simulink model "VCM20_TCon"  (R2021b)
settings: Solver=ode1  StartTime=0.0  StopTime=Inf  FixedStep=0.001  RelTol=1e-3
PostLoadFcn:
  | , if any(exist('dsrtsu_mdlpostloadfcn', 'file') ~= 0), dsrtsu_mdlpostloadfcn('Execute', bdroot); end,
values from neighbouring files (symbols this model uses):
  gear_f = 14.45    [VehicleParamsFEM20_Gear17.m]
  Rwf = 18*(25.4/1000)/2    (= 0.2286)    [VehicleParamsFEM20_Gear17.m]
libraries: rtican x62, dspstat3 x9, simulink x8, rti1401lib_dio_type4 x4, rti1401lib_adc_type4 x4
(part 5 of 12)

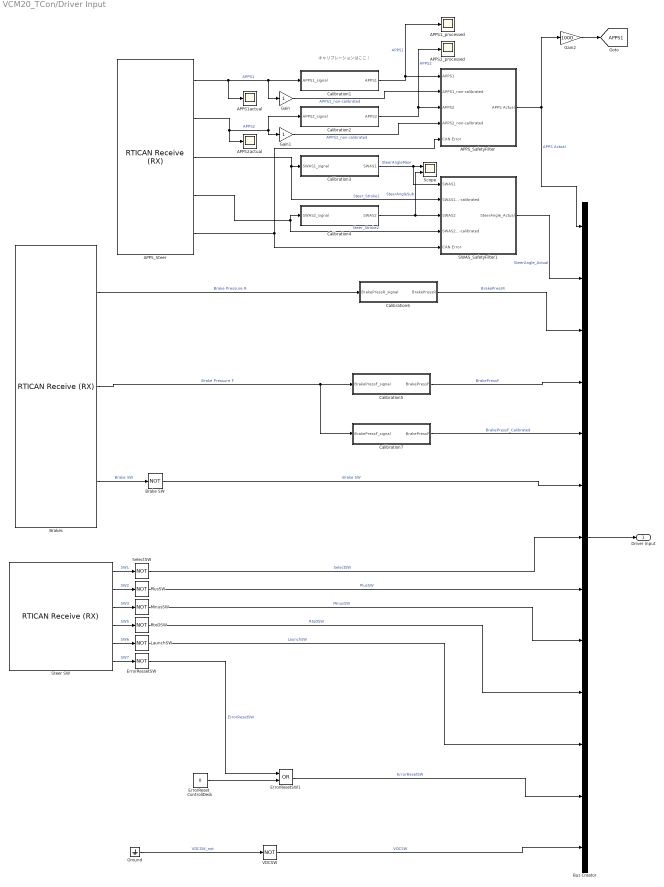
== system VCM20_TCon/Driver Input ==
  note: キャリブレーションはここ！
  APPS1_processed : Scope
  APPS1actual : Scope
  APPS2_processed : Scope
  APPS2actual : Scope
  APPS_SafetyFilter : Subsystem
  APPS_Steer : rtican/RTICAN Receive (RX)   Reserved1=[]  Reserved2=[]  Reserved3=[]  Reserved4=[]  SfcnMessage=[]  Msg_Struct=[]  BoardTypeNo=[]  BoardNo=[]  ChannelNo=[]  Parameters=[]  DialogFcn=[]  UnitName=[]  Revision=[]  UnitValues=[]  DSProperties=struct('RTI',struct('Version',uint32(5),'BlockType',struct('isSLSource',uint8(1),'isSLSink',uint8(1),'isHWSource',uint8(0),'isHWSink',uint8(0),'isSetup',uint8(0),'isInline',uint8(1),'isNonInline',uint8(0),'isInterrupt',uint8(0),'isChannelwise',uint8(0)),'IOBoardType','RTICAN','UnitType','MESSAGE','Identifier','RX','DialogType','MSVC','BlockSet','RTICAN','SlaveProcessor','CAN'))  RTIBlockInterface=struct('OutputPortsWidth',int32([1 1 1 1 1]),'OutputPortsActive',[1 1 1 1 1],'OutputPortsName',{{'APPS1','APPS2','Steer_Stroke1','Steer_Stroke2',['RX status']}},'OutputPortsDataType',{{'SS_DOUBLE','SS_DOUBLE','SS_DOUBLE','SS_DOUBLE','SS_DOUBLE'}},'OutputPortsLabel',{{'APPS1','APPS2','Steer_Stroke1','Steer_Stroke2',''}},'OutputPortsLabelMode','ON','InputPortsWidth',int32(0),'InputPortsActive',0,'DialogFcn','rtican_message_interface_gui','BlockDisplay',{{'','center'}},'IconTransparency','on','ParameterTunableNames',{{}},'InitLevel',3,'BlockName',struct('Token',{{'APPS_Steer'}}),'SampleTime',{{0.01}},'TriggerPort',{{'none'}},'EnablePort',{{'none'}})  RTIBlockParameters=struct('BoardTypeNo',{{1,'OFF',[]}},'BoardNo',{{3,'ON',[1 16]}},'ChannelNo',{{2,'ON',[1 2]}},'Parameters',{{struct('DataFileSupport',struct('DataFileSelectedMaster',0,'DataFileSelectedLocal',0,'DataFileName',['<no datafile support>|'],'DataFileDate','','SelectedFile',['<no file selected>']),'Options',struct('StatusSelected',1,'TimeSelected',0,'DeltaTimeSelected',0,'BytePortSelected',0,'MessageLengthSelected',0,'TriggerPort',struct('Selected',0,'TriggerType',0),'UserCoding',struct('Selected',0,'InterfaceFile','UserDecodingFile','FcnName','UserDecodeFcn','InportSelected',0,'InportWidth',1,'OutportSelected',0,'OutportWidth',1),'EnablePortSelected',0,'SignalOnPortnameSelected',1,'UseRXService',0),'Message',struct('MsgOnBlocknameSelected',1,'MsgName','APPS_Steer','MsgIdFormat',0,'MsgId',513,'MsgLength',8,'NumSignals',4,'SampleTime',0.01,'Signal',struct('SgnName',{'APPS1','APPS2','Steer_Stroke1','Steer_Stroke2'},'SgnStartBit',{0,16,32,48},'SgnLength',{16,16,16,16},'SgnType',{0,0,0,0},'ModeValue',{-1,-1,-1,-1},'DataType',{0,0,0,0},'ByteLayout',{0,0,0,0},'Factor',{1,1,1,1},'Offset',{0,0,0,0},'SgnComment',{{''},{''},{''},{''}},'SgnUnit',{'','','',''},'Min',{0,0,0,0},'Max',{0,0,0,0},'SLDataType',{'SS_DOUBLE','SS_DOUBLE','SS_DOUBLE','SS_DOUBLE'}),'MsgIdNumFormat',1,'MsgComment',{{''}}),'Version',1.2,'general',struct('isFromLib',0)),'OFF',[]}},'GroupId',{{struct('Group',{{'RTICAN'}},'No',6,'Behavior',{{'NAMECHANGE'}},'BlockType',{{'SINK'}},'NameChangeFlag',0),'OFF',[]}},'SFcnRTICANMessage',{{struct('MsgType','RX','SFcnPortType','Scalar','MsgName','APPS_Steer','MsgIdFormat','STD','MsgId',513,'MsgLength',8,'NumSignals',4,'SampleTime',0.01,'Signal',struct('SgnName',{'APPS1','APPS2','Steer_Stroke1','Steer_Stroke2'},'SgnStartBit',{0,16,32,48},'SgnLength',{16,16,16,16},'SgnType',{'standard','standard','standard','standard'},'ModeValue',{-1,-1,-1,-1},'DataType',{['unsigned int'],['unsigned int'],['unsigned int'],['unsigned int']},'ByteLayout',{['little endian'],['little endian'],['little endian'],['little endian']},'Factor',{1,1,1,1},'Offset',{0,0,0,0},'SLDataType',{'SS_DOUBLE','SS_DOUBLE','SS_DOUBLE','SS_DOUBLE'}),'StatusSelected','yes','TimeSelected','no','DeltaTimeSelected','no','BytePortSelected','no','MessageLengthSelected','no','TriggerPort',struct('Selected','no','TriggerType',0),'UserCoding',struct('Selected','no','InterfaceFile','UserDecodingFile','FcnName','UserDecodeFcn','InportSelected','no','InportWidth',1,'OutportSelected','no','OutportWidth',1),'EnablePortSelected','no','UseRXService','no','BoardType','DS1','BoardNo',3,'ControllerNo',2),'OFF',[]}},'TLCFileName',{{'rtican_rx_message','OFF',[]}})  RTISFcnParameters=struct('SFcnRTICANMessage','struct','TLCFileName','char')  RTIBlockParaDefault=struct('BoardTypeNo',4302,'BoardNo',1,'ChannelNo',1,'Parameters',struct('DataFileSupport',struct('DataFileSelectedMaster',0,'DataFileSelectedLocal',0,'DataFileName','','DataFileDate','','SelectedFile',['<no file selected>']),'Options',struct('StatusSelected',1,'TimeSelected',1,'DeltaTimeSelected',1,'BytePortSelected',0,'MessageLengthSelected',0,'TriggerPort',struct('Selected',0,'TriggerType','rising'),'UserCoding',struct('Selected',0,'InterfaceFile','UserDecodingFile','FcnName','UserDecodeFcn','InportSelected',0,'InportWidth',1,'OutportSelected',0,'OutportWidth',1),'EnablePortSelected',0,'SignalOnPortnameSelected',1,'UseRXService',0),'Message',struct('MsgOnBlocknameSelected',0,'MsgName',['RX Message'],'MsgIdFormat',0,'MsgId',100,'MsgLength',8,'NumSignals',1,'SampleTime',-1,'Signal',struct('SgnName',['RX signal'],'SgnStartBit',0,'SgnLength',8,'SgnType',0,'ModeValue',-1,'DataType',0,'SLDataType','SS_DOUBLE','ByteLayout',0,'Factor',1,'Offset',0,'Min',0,'Max',255,'SgnComment',{{}},'SgnUnit',''),'MsgIdNumFormat',0,'MsgComment',{{''}}),'Version',1.2,'general',struct('isFromLib',1)),'GroupId',struct('Group',{{'RTICAN'}},'No',1,'Behavior',{{'NAMECHANGE'}},'BlockType',{{'SINK'}},'NameChangeFlag',0),'SFcnRTICANMessage',struct('MsgType','RX','MsgName',['RX Message'],'MsgIdFormat','STD','MsgId',100,'MsgLength',8,'NumSignals',1,'SampleTime',-1,'Signal',struct('SgnName',['RX signal'],'SgnStartBit',0,'SgnLength',8,'SgnType','standard','ModeValue',-1,'DataType',['unsigned int'],'ByteLayout',['little endian'],'SLDataType','SS_DOUBLE','Factor',1,'Offset',0),'StatusSelected','yes','TimeSelected','yes','DeltaTimeSelected','yes','BytePortSelected','no','MessageLengthSelected','no','EnablePortSelected','no','UserCoding',struct('Selected','no','InterfaceFile','UserDecodingFile','FcnName','UserDecodeFcn','InportSelected','no','InportWidth',1,'OutportSelected','no','OutportWidth',1),'TriggerPort',struct('Selected','no','TriggerType','rising'),'UseRXService','no','BoardType','DS4302','BoardNo',1,'ControllerNo',1,'SFcnPortType','Scalar'),'TLCFileName','rtican_rx_message')
      settings: AttributesFormatString=Group Id: RTICAN6\n  SourceProductName=dSPACE RTI CAN Blockset
  Brake SW : Logic  Operator=NOT  IconShape=distinctive  AllPortsSameDT=off  OutDataTypeStr=boolean
  Brakes : rtican/RTICAN Receive (RX)   Reserved1=[]  Reserved2=[]  Reserved3=[]  Reserved4=[]  SfcnMessage=[]  Msg_Struct=[]  BoardTypeNo=[]  BoardNo=[]  ChannelNo=[]  Parameters=[]  DialogFcn=[]  UnitName=[]  Revision=[]  UnitValues=[]  DSProperties=struct('RTI',struct('Version',uint32(5),'BlockType',struct('isSLSource',uint8(1),'isSLSink',uint8(1),'isHWSource',uint8(0),'isHWSink',uint8(0),'isSetup',uint8(0),'isInline',uint8(1),'isNonInline',uint8(0),'isInterrupt',uint8(0),'isChannelwise',uint8(0)),'IOBoardType','RTICAN','UnitType','MESSAGE','Identifier','RX','DialogType','MSVC','BlockSet','RTICAN','SlaveProcessor','CAN'))  RTIBlockInterface=struct('OutputPortsWidth',int32([1 1 1]),'OutputPortsActive',[1 1 1],'OutputPortsName',{{['Brake Pressure R'],['Brake Pressure F'],['Brake SW']}},'OutputPortsDataType',{{'SS_DOUBLE','SS_DOUBLE','SS_DOUBLE'}},'OutputPortsLabel',{{['Brake Pressure R'],['Brake Pressure F'],['Brake SW']}},'OutputPortsLabelMode','ON','InputPortsWidth',int32(0),'InputPortsActive',0,'DialogFcn','rtican_message_interface_gui','BlockDisplay',{{'','center'}},'IconTransparency','on','ParameterTunableNames',{{}},'InitLevel',3,'BlockName',struct('Token',{{'Brakes'}}),'SampleTime',{{0.01}},'TriggerPort',{{'none'}},'EnablePort',{{'none'}})  RTIBlockParameters=struct('BoardTypeNo',{{1,'OFF',[]}},'BoardNo',{{3,'ON',[1 16]}},'ChannelNo',{{2,'ON',[1 2]}},'Parameters',{{struct('DataFileSupport',struct('DataFileSelectedMaster',0,'DataFileSelectedLocal',0,'DataFileName',['<no datafile support>|'],'DataFileDate','','SelectedFile',['<no file selected>']),'Options',struct('StatusSelected',0,'TimeSelected',0,'DeltaTimeSelected',0,'BytePortSelected',0,'MessageLengthSelected',0,'TriggerPort',struct('Selected',0,'TriggerType',0),'UserCoding',struct('Selected',0,'InterfaceFile','UserDecodingFile','FcnName','UserDecodeFcn','InportSelected',0,'InportWidth',1,'OutportSelected',0,'OutportWidth',1),'EnablePortSelected',0,'SignalOnPortnameSelected',1,'UseRXService',0),'Message',struct('MsgOnBlocknameSelected',1,'MsgName','Brakes','MsgIdFormat',0,'MsgId',514,'MsgLength',8,'NumSignals',3,'SampleTime',0.01,'Signal',struct('SgnName',{['Brake Pressure R'],['Brake Pressure F'],['Brake SW']},'SgnStartBit',{0,16,32},'SgnLength',{16,16,8},'SgnType',{0,0,0},'ModeValue',{-1,-1,-1},'DataType',{0,0,0},'ByteLayout',{0,0,0},'Factor',{1,1,1},'Offset',{0,0,0},'SgnComment',{{''},{''},{''}},'SgnUnit',{'','',''},'Min',{0,0,0},'Max',{0,0,0},'SLDataType',{'SS_DOUBLE','SS_DOUBLE','SS_DOUBLE'}),'MsgIdNumFormat',1,'MsgComment',{{''}}),'Version',1.2,'general',struct('isFromLib',0)),'OFF',[]}},'GroupId',{{struct('Group',{{'RTICAN'}},'No',6,'Behavior',{{'NAMECHANGE'}},'BlockType',{{'SINK'}},'NameChangeFlag',0),'OFF',[]}},'SFcnRTICANMessage',{{struct('MsgType','RX','SFcnPortType','Scalar','MsgName','Brakes','MsgIdFormat','STD','MsgId',514,'MsgLength',8,'NumSignals',3,'SampleTime',0.01,'Signal',struct('SgnName',{['Brake Pressure R'],['Brake Pressure F'],['Brake SW']},'SgnStartBit',{0,16,32},'SgnLength',{16,16,8},'SgnType',{'standard','standard','standard'},'ModeValue',{-1,-1,-1},'DataType',{['unsigned int'],['unsigned int'],['unsigned int']},'ByteLayout',{['little endian'],['little endian'],['little endian']},'Factor',{1,1,1},'Offset',{0,0,0},'SLDataType',{'SS_DOUBLE','SS_DOUBLE','SS_DOUBLE'}),'StatusSelected','no','TimeSelected','no','DeltaTimeSelected','no','BytePortSelected','no','MessageLengthSelected','no','TriggerPort',struct('Selected','no','TriggerType',0),'UserCoding',struct('Selected','no','InterfaceFile','UserDecodingFile','FcnName','UserDecodeFcn','InportSelected','no','InportWidth',1,'OutportSelected','no','OutportWidth',1),'EnablePortSelected','no','UseRXService','no','BoardType','DS1','BoardNo',3,'ControllerNo',2),'OFF',[]}},'TLCFileName',{{'rtican_rx_message','OFF',[]}})  RTISFcnParameters=struct('SFcnRTICANMessage','struct','TLCFileName','char')  RTIBlockParaDefault=struct('BoardTypeNo',4302,'BoardNo',1,'ChannelNo',1,'Parameters',struct('DataFileSupport',struct('DataFileSelectedMaster',0,'DataFileSelectedLocal',0,'DataFileName','','DataFileDate','','SelectedFile',['<no file selected>']),'Options',struct('StatusSelected',1,'TimeSelected',1,'DeltaTimeSelected',1,'BytePortSelected',0,'MessageLengthSelected',0,'TriggerPort',struct('Selected',0,'TriggerType','rising'),'UserCoding',struct('Selected',0,'InterfaceFile','UserDecodingFile','FcnName','UserDecodeFcn','InportSelected',0,'InportWidth',1,'OutportSelected',0,'OutportWidth',1),'EnablePortSelected',0,'SignalOnPortnameSelected',1,'UseRXService',0),'Message',struct('MsgOnBlocknameSelected',0,'MsgName',['RX Message'],'MsgIdFormat',0,'MsgId',100,'MsgLength',8,'NumSignals',1,'SampleTime',-1,'Signal',struct('SgnName',['RX signal'],'SgnStartBit',0,'SgnLength',8,'SgnType',0,'ModeValue',-1,'DataType',0,'SLDataType','SS_DOUBLE','ByteLayout',0,'Factor',1,'Offset',0,'Min',0,'Max',255,'SgnComment',{{}},'SgnUnit',''),'MsgIdNumFormat',0,'MsgComment',{{''}}),'Version',1.2,'general',struct('isFromLib',1)),'GroupId',struct('Group',{{'RTICAN'}},'No',1,'Behavior',{{'NAMECHANGE'}},'BlockType',{{'SINK'}},'NameChangeFlag',0),'SFcnRTICANMessage',struct('MsgType','RX','MsgName',['RX Message'],'MsgIdFormat','STD','MsgId',100,'MsgLength',8,'NumSignals',1,'SampleTime',-1,'Signal',struct('SgnName',['RX signal'],'SgnStartBit',0,'SgnLength',8,'SgnType','standard','ModeValue',-1,'DataType',['unsigned int'],'ByteLayout',['little endian'],'SLDataType','SS_DOUBLE','Factor',1,'Offset',0),'StatusSelected','yes','TimeSelected','yes','DeltaTimeSelected','yes','BytePortSelected','no','MessageLengthSelected','no','EnablePortSelected','no','UserCoding',struct('Selected','no','InterfaceFile','UserDecodingFile','FcnName','UserDecodeFcn','InportSelected','no','InportWidth',1,'OutportSelected','no','OutportWidth',1),'TriggerPort',struct('Selected','no','TriggerType','rising'),'UseRXService','no','BoardType','DS4302','BoardNo',1,'ControllerNo',1,'SFcnPortType','Scalar'),'TLCFileName','rtican_rx_message')
      settings: AttributesFormatString=Group Id: RTICAN6\n  SourceProductName=dSPACE RTI CAN Blockset
  Bus Creator : BusCreator  Inputs=13
  Calibration1 : Subsystem
  Calibration2 : Subsystem
  Calibration3 : Subsystem
  Calibration4 : Subsystem
  Calibration5 : Subsystem
  Calibration6 : Subsystem
  Calibration7 : Subsystem
  ErrorResetSW1 : Logic  Operator=OR  AllPortsSameDT=off  OutDataTypeStr=boolean
  ErrorReset_ControllDesk : Constant  Value=0
  ErrorRessetSW : Logic  Operator=NOT  IconShape=distinctive  AllPortsSameDT=off  OutDataTypeStr=boolean
  Gain : Gain
  Gain1 : Gain
  Gain2 : Gain  Gain=1000
  Ground : Ground
  LaunchSW : Logic  Operator=NOT  IconShape=distinctive  AllPortsSameDT=off  OutDataTypeStr=boolean
  MinusSW : Logic  Operator=NOT  IconShape=distinctive  AllPortsSameDT=off  OutDataTypeStr=boolean
  PlusSW : Logic  Operator=NOT  IconShape=distinctive  AllPortsSameDT=off  OutDataTypeStr=boolean
  RtoDSW : Logic  Operator=NOT  IconShape=distinctive  AllPortsSameDT=off  OutDataTypeStr=boolean
  SWAS_SafetyFilter1 : Subsystem
  Scope : Scope  NumInputPorts=2
  SelectSW : Logic  Operator=NOT  IconShape=distinctive  AllPortsSameDT=off  OutDataTypeStr=boolean
  Steer SW : rtican/RTICAN Receive (RX)   Reserved1=[]  Reserved2=[]  Reserved3=[]  Reserved4=[]  SfcnMessage=[]  Msg_Struct=[]  BoardTypeNo=[]  BoardNo=[]  ChannelNo=[]  Parameters=[]  DialogFcn=[]  UnitName=[]  Revision=[]  UnitValues=[]  DSProperties=struct('RTI',struct('Version',uint32(5),'BlockType',struct('isSLSource',uint8(1),'isSLSink',uint8(1),'isHWSource',uint8(0),'isHWSink',uint8(0),'isSetup',uint8(0),'isInline',uint8(1),'isNonInline',uint8(0),'isInterrupt',uint8(0),'isChannelwise',uint8(0)),'IOBoardType','RTICAN','UnitType','MESSAGE','Identifier','RX','DialogType','MSVC','BlockSet','RTICAN','SlaveProcessor','CAN'))  RTIBlockInterface=struct('OutputPortsWidth',int32([1 1 1 1 1 1]),'OutputPortsActive',[1 1 1 1 1 1],'OutputPortsName',{{'SW1','SW2','SW3','SW5','SW6','SW7'}},'OutputPortsDataType',{{'SS_DOUBLE','SS_DOUBLE','SS_DOUBLE','SS_DOUBLE','SS_DOUBLE','SS_DOUBLE'}},'OutputPortsLabel',{{'SW1','SW2','SW3','SW5','SW6','SW7'}},'OutputPortsLabelMode','ON','InputPortsWidth',int32(0),'InputPortsActive',0,'DialogFcn','rtican_message_interface_gui','BlockDisplay',{{'','center'}},'IconTransparency','on','ParameterTunableNames',{{}},'InitLevel',3,'BlockName',struct('Token',{{'Brakes'}}),'SampleTime',{{0.1}},'TriggerPort',{{'none'}},'EnablePort',{{'none'}})  RTIBlockParameters=struct('BoardTypeNo',{{1,'OFF',[]}},'BoardNo',{{1,'ON',[1 16]}},'ChannelNo',{{1,'ON',[1 2]}},'Parameters',{{struct('DataFileSupport',struct('DataFileSelectedMaster',0,'DataFileSelectedLocal',0,'DataFileName',['<no datafile support>|'],'DataFileDate','','SelectedFile',['<no file selected>']),'Options',struct('StatusSelected',0,'TimeSelected',0,'DeltaTimeSelected',0,'BytePortSelected',0,'MessageLengthSelected',0,'TriggerPort',struct('Selected',0,'TriggerType',0),'UserCoding',struct('Selected',0,'InterfaceFile','UserDecodingFile','FcnName','UserDecodeFcn','InportSelected',0,'InportWidth',1,'OutportSelected',0,'OutportWidth',1),'EnablePortSelected',0,'SignalOnPortnameSelected',1,'UseRXService',0),'Message',struct('MsgOnBlocknameSelected',1,'MsgName',['Steer SW'],'MsgIdFormat',0,'MsgId',512,'MsgLength',1,'NumSignals',6,'SampleTime',0.1,'Signal',struct('SgnName',{'SW1','SW2','SW3','SW5','SW6','SW7'},'SgnStartBit',{0,1,2,3,4,5},'SgnLength',{1,1,1,1,1,1},'SgnType',{0,0,0,0,0,0},'ModeValue',{-1,-1,-1,-1,-1,-1},'DataType',{0,0,0,0,0,0},'ByteLayout',{0,0,0,0,0,0},'Factor',{1,1,1,1,1,1},'Offset',{0,0,0,0,0,0},'SgnComment',{{''},{''},{''},{''},{''},{''}},'SgnUnit',{'','','','','',''},'Min',{0,0,0,0,0,0},'Max',{0,0,0,0,0,0},'SLDataType',{'SS_DOUBLE','SS_DOUBLE','SS_DOUBLE','SS_DOUBLE','SS_DOUBLE','SS_DOUBLE'}),'MsgIdNumFormat',1,'MsgComment',{{''}}),'Version',1.2,'general',struct('isFromLib',0)),'OFF',[]}},'GroupId',{{struct('Group',{{'RTICAN'}},'No',1,'Behavior',{{'NAMECHANGE'}},'BlockType',{{'SINK'}},'NameChangeFlag',0),'OFF',[]}},'SFcnRTICANMessage',{{struct('MsgType','RX','SFcnPortType','Scalar','MsgName',['Steer SW'],'MsgIdFormat','STD','MsgId',512,'MsgLength',1,'NumSignals',6,'SampleTime',0.1,'Signal',struct('SgnName',{'SW1','SW2','SW3','SW5','SW6','SW7'},'SgnStartBit',{0,1,2,3,4,5},'SgnLength',{1,1,1,1,1,1},'SgnType',{'standard','standard','standard','standard','standard','standard'},'ModeValue',{-1,-1,-1,-1,-1,-1},'DataType',{['unsigned int'],['unsigned int'],['unsigned int'],['unsigned int'],['unsigned int'],['unsigned int']},'ByteLayout',{['little endian'],['little endian'],['little endian'],['little endian'],['little endian'],['little endian']},'Factor',{1,1,1,1,1,1},'Offset',{0,0,0,0,0,0},'SLDataType',{'SS_DOUBLE','SS_DOUBLE','SS_DOUBLE','SS_DOUBLE','SS_DOUBLE','SS_DOUBLE'}),'StatusSelected','no','TimeSelected','no','DeltaTimeSelected','no','BytePortSelected','no','MessageLengthSelected','no','TriggerPort',struct('Selected','no','TriggerType',0),'UserCoding',struct('Selected','no','InterfaceFile','UserDecodingFile','FcnName','UserDecodeFcn','InportSelected','no','InportWidth',1,'OutportSelected','no','OutportWidth',1),'EnablePortSelected','no','UseRXService','no','BoardType','DS1','BoardNo',1,'ControllerNo',1),'OFF',[]}},'TLCFileName',{{'rtican_rx_message','OFF',[]}})  RTISFcnParameters=struct('SFcnRTICANMessage','struct','TLCFileName','char')  RTIBlockParaDefault=struct('BoardTypeNo',4302,'BoardNo',1,'ChannelNo',1,'Parameters',struct('DataFileSupport',struct('DataFileSelectedMaster',0,'DataFileSelectedLocal',0,'DataFileName','','DataFileDate','','SelectedFile',['<no file selected>']),'Options',struct('StatusSelected',1,'TimeSelected',1,'DeltaTimeSelected',1,'BytePortSelected',0,'MessageLengthSelected',0,'TriggerPort',struct('Selected',0,'TriggerType','rising'),'UserCoding',struct('Selected',0,'InterfaceFile','UserDecodingFile','FcnName','UserDecodeFcn','InportSelected',0,'InportWidth',1,'OutportSelected',0,'OutportWidth',1),'EnablePortSelected',0,'SignalOnPortnameSelected',1,'UseRXService',0),'Message',struct('MsgOnBlocknameSelected',0,'MsgName',['RX Message'],'MsgIdFormat',0,'MsgId',100,'MsgLength',8,'NumSignals',1,'SampleTime',-1,'Signal',struct('SgnName',['RX signal'],'SgnStartBit',0,'SgnLength',8,'SgnType',0,'ModeValue',-1,'DataType',0,'SLDataType','SS_DOUBLE','ByteLayout',0,'Factor',1,'Offset',0,'Min',0,'Max',255,'SgnComment',{{}},'SgnUnit',''),'MsgIdNumFormat',0,'MsgComment',{{''}}),'Version',1.2,'general',struct('isFromLib',1)),'GroupId',struct('Group',{{'RTICAN'}},'No',1,'Behavior',{{'NAMECHANGE'}},'BlockType',{{'SINK'}},'NameChangeFlag',0),'SFcnRTICANMessage',struct('MsgType','RX','MsgName',['RX Message'],'MsgIdFormat','STD','MsgId',100,'MsgLength',8,'NumSignals',1,'SampleTime',-1,'Signal',struct('SgnName',['RX signal'],'SgnStartBit',0,'SgnLength',8,'SgnType','standard','ModeValue',-1,'DataType',['unsigned int'],'ByteLayout',['little endian'],'SLDataType','SS_DOUBLE','Factor',1,'Offset',0),'StatusSelected','yes','TimeSelected','yes','DeltaTimeSelected','yes','BytePortSelected','no','MessageLengthSelected','no','EnablePortSelected','no','UserCoding',struct('Selected','no','InterfaceFile','UserDecodingFile','FcnName','UserDecodeFcn','InportSelected','no','InportWidth',1,'OutportSelected','no','OutportWidth',1),'TriggerPort',struct('Selected','no','TriggerType','rising'),'UseRXService','no','BoardType','DS4302','BoardNo',1,'ControllerNo',1,'SFcnPortType','Scalar'),'TLCFileName','rtican_rx_message')
      settings: AttributesFormatString=Group Id: RTICAN1\n  SourceProductName=dSPACE RTI CAN Blockset
  VDCSW : Logic  Operator=NOT  AllPortsSameDT=off  OutDataTypeStr=boolean
  Driver Input : Outport  VectorParamsAs1DForOutWhenUnconnected=off
  tag scope: APPS1=global
  wires:
  APPS_Steer/1 -> APPS1actual/1, Gain/1, Calibration1/1(APPS1_signal)  "APPS1"
  APPS_Steer/2 -> APPS2actual/1, Calibration2/1(APPS2_signal), Gain1/1  "APPS2"
  APPS_Steer/3 -> SWAS_SafetyFilter1/2(SWAS1_non-calibrated), Calibration3/1(SWAS1_signal)  "Steer_Stroke1"
  APPS_Steer/4 -> Calibration4/1(SWAS2_signal), SWAS_SafetyFilter1/4(SWAS2_non-calibrated)  "Steer_Stroke2"
  Brakes/2 -> Calibration7/1(BrakePressF_signal), Calibration5/1(BrakePressF_signal)  "Brake Pressure F"
  Brakes/1 -> Calibration6/1(BrakePressR_signal)  "Brake Pressure R"
  Calibration3/1(SWAS1) -> SWAS_SafetyFilter1/1(SWAS1), Scope/1  "SteerAngleMain"
  Calibration4/1(SWAS2) -> Scope/2, SWAS_SafetyFilter1/3(SWAS2)  "SteerAngleSub"
  Calibration5/1(BrakePressF) -> Bus Creator/4  "BrakePressF"
  Calibration6/1(BrakePressR) -> Bus Creator/3  "BrakePressR"
  Bus Creator/1 -> Driver Input/1
  RtoDSW/1 -> Bus Creator/10  "RtoDSW"
  LaunchSW/1 -> Bus Creator/11  "LaunchSW"
  ErrorResetSW1/1 -> Bus Creator/12  "ErrorResetSW"
  VDCSW/1 -> Bus Creator/13  "VDCSW"
  Brake SW/1 -> Bus Creator/6  "Brake SW"
  Ground/1 -> VDCSW/1  "VDCSW_not"
  ErrorRessetSW/1 -> ErrorResetSW1/1  "ErrorResetSW"
  ErrorReset_ControllDesk/1 -> ErrorResetSW1/2
  Calibration1/1(APPS1) -> APPS_SafetyFilter/1(APPS1), APPS1_processed/1  "APPS1"
  Calibration2/1(APPS2) -> APPS_SafetyFilter/3(APPS2), APPS2_processed/1  "APPS2"
  Gain/1 -> APPS_SafetyFilter/2(APPS1_non-calibrated)  "APPS1_non-calibrated"
  Gain1/1 -> APPS_SafetyFilter/4(APPS2_non-calibrated)  "APPS2_non-calibrated"
  APPS_SafetyFilter/1(APPS Actual) -> Gain2/1, Bus Creator/1  "APPS Actual"
  SWAS_SafetyFilter1/1(SteerAngle_Actual) -> Bus Creator/2  "SteerAngle_Actual"
  Steer SW/1 -> SelectSW/1  "SW1"
  Steer SW/2 -> PlusSW/1  "SW2"
  Steer SW/3 -> MinusSW/1  "SW3"
  SelectSW/1 -> Bus Creator/7  "SelectSW"
  PlusSW/1 -> Bus Creator/8  "PlusSW"
  MinusSW/1 -> Bus Creator/9  "MinusSW"
  Steer SW/4 -> RtoDSW/1  "SW5"
  Steer SW/5 -> LaunchSW/1  "SW6"
  Steer SW/6 -> ErrorRessetSW/1  "SW7"
  Brakes/3 -> Brake SW/1  "Brake SW"
  Gain2/1 -> [APPS1]
  APPS_Steer/5 -> APPS_SafetyFilter/5(CAN Error), SWAS_SafetyFilter1/5(CAN Error)
  Calibration7/1(BrakePressF) -> Bus Creator/5  "BrakePressF_Calibrated"

== system VCM20_TCon/From relay board ==
  AMS_shutdownsig : rti1401lib_dio_type4/DIO_TYPE4_BIT_IN_CH_BL1  DSProperties=struct('RTI',struct('Version',uint32(1),'BlockType',struct('isSLSource',uint8(1),'isSLSink',uint8(0),'isHWSource',uint8(1),'isHWSink',uint8(0),'isSetup',uint8(0),'isInline',uint8(1),'isNonInline',uint8(0),'isInterrupt',uint8(0),'isChannelwise',uint8(1)),'IOBoardType',{{'DS1401','STD','DIOT4'}},'UnitType','BIT','Identifier','BITINCH','DialogType','ML','BlockSet','NONE','SlaveProcessor','NONE'))  RTIBlockInterface=struct('OutputPortsWidth',int32(1),'OutputPortsDataType',{{'SS_BOOLEAN'}},'OutputPortsActive',1,'OutputPortsName',{{'Out'}},'BlockDisplay',{{['DIO TP4 BIT IN\n Channelwise\nModule: 1\nPort: 1\nChannel: 5'],'center'}},'IconTransparency','on','InitLevel',3,'DialogFcn','rti1401stddiot4bitinchgui','BlockName',struct('Token',{{'DIO_TYPE4_BIT_IN_CH_BL1'}}))  RTIBlockParameters=struct('ModuleNo',{{1,'OFF',[1 16]}},'PortNo',{{1,'OFF',[1 2]}},'ChannelNo',{{5,'OFF',[1 16]}},'TLCFileName',{{'rti1401dio_t4_bit_in_ch','OFF',[]}},'EnableInterrupt',{{0,'OFF',[0 1]}},'TriggerEdgeType',{{1,'OFF',[1 3]}})  RTISFcnParameters=struct('ModuleNo','int32','PortNo','int16','ChannelNo','int16','TLCFileName','char','EnableInterrupt','int16','TriggerEdgeType','int32')  RTIBlockParaDefault=struct('ModuleNo',1,'PortNo',1,'ChannelNo',1,'TLCFileName','rti1401dio_t4_bit_in_ch','EnableInterrupt',0,'TriggerEdgeType',1)
  BSPD_shutdownsig : rti1401lib_dio_type4/DIO_TYPE4_BIT_IN_CH_BL1  DSProperties=struct('RTI',struct('Version',uint32(1),'BlockType',struct('isSLSource',uint8(1),'isSLSink',uint8(0),'isHWSource',uint8(1),'isHWSink',uint8(0),'isSetup',uint8(0),'isInline',uint8(1),'isNonInline',uint8(0),'isInterrupt',uint8(0),'isChannelwise',uint8(1)),'IOBoardType',{{'DS1401','STD','DIOT4'}},'UnitType','BIT','Identifier','BITINCH','DialogType','ML','BlockSet','NONE','SlaveProcessor','NONE'))  RTIBlockInterface=struct('OutputPortsWidth',int32(1),'OutputPortsDataType',{{'SS_BOOLEAN'}},'OutputPortsActive',1,'OutputPortsName',{{'Out'}},'BlockDisplay',{{['DIO TP4 BIT IN\n Channelwise\nModule: 1\nPort: 1\nChannel: 15'],'center'}},'IconTransparency','on','InitLevel',3,'DialogFcn','rti1401stddiot4bitinchgui','BlockName',struct('Token',{{'DIO_TYPE4_BIT_IN_CH_BL1'}}))  RTIBlockParameters=struct('ModuleNo',{{1,'OFF',[1 16]}},'PortNo',{{1,'OFF',[1 2]}},'ChannelNo',{{15,'OFF',[1 16]}},'TLCFileName',{{'rti1401dio_t4_bit_in_ch','OFF',[]}},'EnableInterrupt',{{0,'OFF',[0 1]}},'TriggerEdgeType',{{1,'OFF',[1 3]}})  RTISFcnParameters=struct('ModuleNo','int32','PortNo','int16','ChannelNo','int16','TLCFileName','char','EnableInterrupt','int16','TriggerEdgeType','int32')  RTIBlockParaDefault=struct('ModuleNo',1,'PortNo',1,'ChannelNo',1,'TLCFileName','rti1401dio_t4_bit_in_ch','EnableInterrupt',0,'TriggerEdgeType',1)
  Bus Creator : BusCreator  Inputs=3
  IMD_shutdownsig : rti1401lib_dio_type4/DIO_TYPE4_BIT_IN_CH_BL1  DSProperties=struct('RTI',struct('Version',uint32(1),'BlockType',struct('isSLSource',uint8(1),'isSLSink',uint8(0),'isHWSource',uint8(1),'isHWSink',uint8(0),'isSetup',uint8(0),'isInline',uint8(1),'isNonInline',uint8(0),'isInterrupt',uint8(0),'isChannelwise',uint8(1)),'IOBoardType',{{'DS1401','STD','DIOT4'}},'UnitType','BIT','Identifier','BITINCH','DialogType','ML','BlockSet','NONE','SlaveProcessor','NONE'))  RTIBlockInterface=struct('OutputPortsWidth',int32(1),'OutputPortsDataType',{{'SS_BOOLEAN'}},'OutputPortsActive',1,'OutputPortsName',{{'Out'}},'BlockDisplay',{{['DIO TP4 BIT IN\n Channelwise\nModule: 1\nPort: 1\nChannel: 10'],'center'}},'IconTransparency','on','InitLevel',3,'DialogFcn','rti1401stddiot4bitinchgui','BlockName',struct('Token',{{'DIO_TYPE4_BIT_IN_CH_BL1'}}))  RTIBlockParameters=struct('ModuleNo',{{1,'OFF',[1 16]}},'PortNo',{{1,'OFF',[1 2]}},'ChannelNo',{{10,'OFF',[1 16]}},'TLCFileName',{{'rti1401dio_t4_bit_in_ch','OFF',[]}},'EnableInterrupt',{{0,'OFF',[0 1]}},'TriggerEdgeType',{{1,'OFF',[1 3]}})  RTISFcnParameters=struct('ModuleNo','int32','PortNo','int16','ChannelNo','int16','TLCFileName','char','EnableInterrupt','int16','TriggerEdgeType','int32')  RTIBlockParaDefault=struct('ModuleNo',1,'PortNo',1,'ChannelNo',1,'TLCFileName','rti1401dio_t4_bit_in_ch','EnableInterrupt',0,'TriggerEdgeType',1)
  shutdownLEDsig : Outport
  wires:
  AMS_shutdownsig/1 -> Bus Creator/1  "AMS_shutdownsig"
  IMD_shutdownsig/1 -> Bus Creator/2  "IMD_shutdownsig"
  BSPD_shutdownsig/1 -> Bus Creator/3  "BSPD_shutdownsig"
  Bus Creator/1 -> shutdownLEDsig/1  "shutdownLEDsig"

== system VCM20_TCon/RTI Data ==
  RTI Data Store : Subsystem  Tag="struct('private',struct('version',struct('dsVer',uint32(2)),'access',struct('modified',['31-Jul-2023 14:24:14'],'type','Model','isPerm',1)),'public',struct('main',struct('data',[]),'sub',struct('name',{{'VCM20_TCon'}},'data',{{struct('TH',struct('thTaskInfo',struct('taskType',{'TIMER','HWINT','TMRINT','SWINT','GLINT'},'tasksNumOf',{1,0,0,0,0},'srcIds',{{'TIMERA'},{},{},{},{}},'taskNames',{{['Timer Task 1']},{},{},{},{}})),'th_tc',struct('dataType','TASK','taskGroupId','','taskGroupList',{{}},'taskSchedulingPolicy','FCFS','taskType','TIMER','blkh',-1,'srcId','TIMERA','srcSgnName',['Timer A interrupt'],'srcCpuName','','taskName',['Timer Task 1  [0.001] s'],'taskNameDisplayExt','','smplTime',0.001,'smplTimeOffs',0,'hasFixedPriority',0,'priority',1,'hasFixedOvc',0,'ovcType',1,'ovcMax',1),'tc_th',struct('dataType','TASK','taskGroupId','','taskGroupList',{{}},'taskSchedulingPolicy','FCFS','taskType','TIMER','blkh',-1,'srcId','TIMERA','srcSgnName',['Timer A interrupt'],'srcCpuName','','taskName',['Timer Task 1  [0.001] s'],'taskNameDisplayExt','','smplTime',0.001,'smplTimeOffs',0,'hasFixedPriority',0,'priority',1,'hasFixedOvc',0,'ovcType',1,'ovcMax',1))}})))"  mask(RTI_DATA_STORE){}
      mask help:
      | RTI Data Store Block. This block is used by RTI to store internal model dependent data. Deleting this block will result in data loss.
      |
      | NEVER DELETE, COPY, OR MODIFY THIS BLOCK!
      mask Help:
      | RTI Data Store Block. This block is used by RTI to store internal model dependent data. Deleting this block will result in data loss.
      | 
      | NEVER DELETE, COPY, OR MODIFY THIS BLOCK!
      mask Display: text(0.5, 0.5, ' ', 'HorizontalAlignment', 'center');
